simulink model "KheperaIV"  (R2020b)
settings: Solver=VariableStepAuto  StartTime=0.0  StopTime=10.0  RelTol=1e-3
undefined symbols (not defined in the file): I, kb, kt, L, La, m, N, r, Ra, Rr
settings Model: Creator=FranciscoJose  LastModifiedBy=FranciscoJose

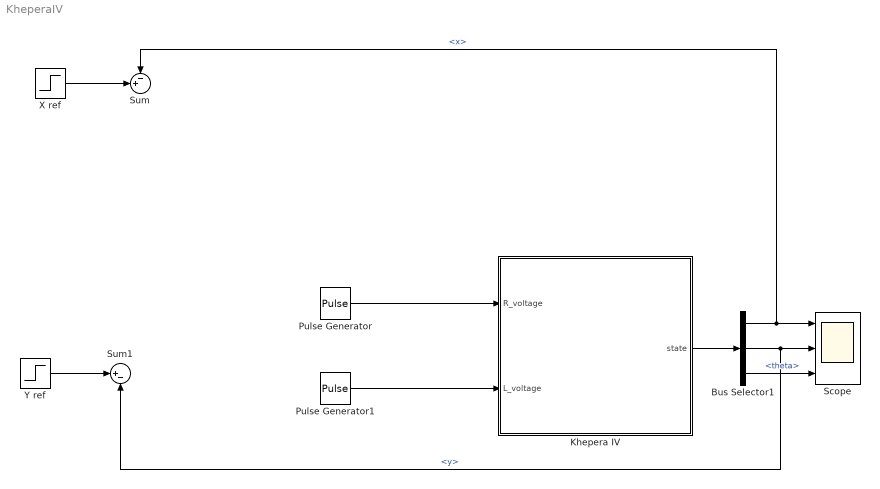
== system KheperaIV ==
  Bus Selector1 : BusSelector  OutputSignals=x,y,theta
  Khepera IV : Subsystem  mask{m=m, kb=kb, kt=kt, N=N, La=La, Ra=Ra, L=L, r=r, I=I, Rr=Rr}
      mask prompts: m "Mass [Kg]"; kb "Back-EMF constant [V/rad/s]"; kt "Torque constant [Nm/A]"; N "Gear ratio"; La "Rotor inductance [H]"; Ra "Terminal resistance [Ohm]"; L "Distance between wheels [m]"; r "Wheels radius [m]"; I "Moment inertia of robot [Kg m^2]"; Rr "Robot radius [m]"
      mask DialogControl DescTextVar Prompt: Khepera IV parameters
      mask Display: image('KheperaIV_icon.png')
  Pulse Generator : DiscretePulseGenerator  PulseType=Time based  Amplitude=6  Period=10  PulseWidth=10
  Pulse Generator1 : DiscretePulseGenerator  PulseType=Time based  Amplitude=-6  Period=10  PulseWidth=10
  Scope : Scope  NumInputPorts=3
  Sum : Sum  Inputs=-+|
  Sum1 : Sum  Inputs=|+-
  X ref : Step  SampleTime=0
  Y ref : Step  SampleTime=0
  wires:
  Khepera IV/1(state) -> Bus Selector1/1
  Bus Selector1/3 -> Scope/3  "<theta>"
  Bus Selector1/2 -> Scope/2, Sum1/2  "<y>"
  Bus Selector1/1 -> Sum/1, Scope/1  "<x>"
  Pulse Generator1/1 -> Khepera IV/2(L_voltage)
  Pulse Generator/1 -> Khepera IV/1(R_voltage)
  X ref/1 -> Sum/2
  Y ref/1 -> Sum1/1

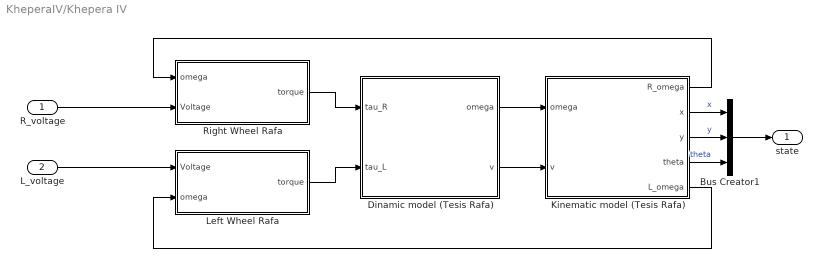
== system KheperaIV/Khepera IV ==
  R_voltage : Inport
  L_voltage : Inport  Port=2
  Bus Creator1 : BusCreator  Inputs=3
  Dinamic model (Tesis Rafa) : Subsystem
  Kinematic model (Tesis Rafa) : Subsystem
  Left Wheel Rafa : Subsystem
  Right Wheel Rafa : Subsystem
  state : Outport
  wires:
  L_voltage/1 -> Left Wheel Rafa/1(Voltage)
  R_voltage/1 -> Right Wheel Rafa/2(Voltage)
  Dinamic model (Tesis Rafa)/1(omega) -> Kinematic model (Tesis Rafa)/1(omega)
  Dinamic model (Tesis Rafa)/2(v) -> Kinematic model (Tesis Rafa)/2(v)
  Left Wheel Rafa/1(torque) -> Dinamic model (Tesis Rafa)/2(tau_L)
  Right Wheel Rafa/1(torque) -> Dinamic model (Tesis Rafa)/1(tau_R)
  Kinematic model (Tesis Rafa)/1(R_omega) -> Right Wheel Rafa/1(omega)
  Kinematic model (Tesis Rafa)/5(L_omega) -> Left Wheel Rafa/2(omega)
  Kinematic model (Tesis Rafa)/2(x) -> Bus Creator1/1  "x"
  Kinematic model (Tesis Rafa)/3(y) -> Bus Creator1/2  "y"
  Kinematic model (Tesis Rafa)/4(theta) -> Bus Creator1/3  "theta"
  Bus Creator1/1 -> state/1

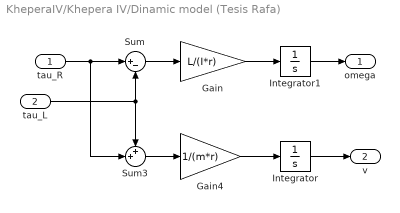
== system KheperaIV/Khepera IV/Dinamic model (Tesis Rafa) ==
  tau_R : Inport
  tau_L : Inport  Port=2
  Gain : Gain  Gain=L/(I*r)
  Gain4 : Gain  Gain=1/(m*r)
  Integrator : Integrator
  Integrator1 : Integrator
  Sum : Sum  Inputs=|+-
  Sum3 : Sum  Inputs=++|
  omega : Outport
  v : Outport  Port=2
  wires:
  Sum/1 -> Gain/1
  Integrator/1 -> v/1
  tau_R/1 -> Sum3/2, Sum/1
  Integrator1/1 -> omega/1
  Gain/1 -> Integrator1/1
  tau_L/1 -> Sum3/1, Sum/2
  Sum3/1 -> Gain4/1
  Gain4/1 -> Integrator/1

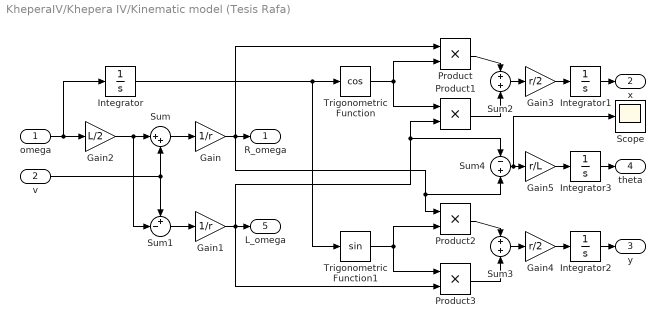
== system KheperaIV/Khepera IV/Kinematic model (Tesis Rafa) ==
  omega : Inport
  v : Inport  Port=2
  Gain : Gain  Gain=1/r
  Gain1 : Gain  Gain=1/r
  Gain2 : Gain  Gain=L/2
  Gain3 : Gain  Gain=r/2
  Gain4 : Gain  Gain=r/2
  Gain5 : Gain  Gain=r/L
  Integrator{,1..3} (4 alike) : Integrator
  Product{,1..3} (4 alike) : Product
  Scope : Scope
  Sum : Sum  Inputs=|++
  Sum1 : Sum  Inputs=+-|
  Sum2 : Sum
  Sum3 : Sum
  Sum4 : Sum  Inputs=-+
  Trigonometric Function : Trigonometry  Operator=cos
  Trigonometric Function1 : Trigonometry
  R_omega : Outport
  x : Outport  Port=2
  y : Outport  Port=3
  theta : Outport  Port=4
  L_omega : Outport  Port=5
  wires:
  Sum/1 -> Gain/1
  Gain2/1 -> Sum1/2, Sum/1
  v/1 -> Sum1/1, Sum/2
  Sum1/1 -> Gain1/1
  omega/1 -> Integrator/1, Gain2/1
  Gain3/1 -> Integrator1/1
  Integrator/1 -> Trigonometric Function1/1, Trigonometric Function/1
  Sum2/1 -> Gain3/1
  Product/1 -> Sum2/1
  Trigonometric Function/1 -> Product/2, Product1/1
  Product1/1 -> Sum2/2
  Gain/1 -> R_omega/1, Sum4/2, Product2/1, Product/1
  Trigonometric Function1/1 -> Product2/2, Product3/1
  Product3/1 -> Sum3/2
  Sum3/1 -> Gain4/1
  Gain1/1 -> L_omega/1, Product3/2, Sum4/1, Product1/2
  Product2/1 -> Sum3/1
  Integrator1/1 -> x/1
  Gain4/1 -> Integrator2/1
  Integrator2/1 -> y/1
  Integrator3/1 -> theta/1
  Gain5/1 -> Integrator3/1
  Sum4/1 -> Scope/1, Gain5/1

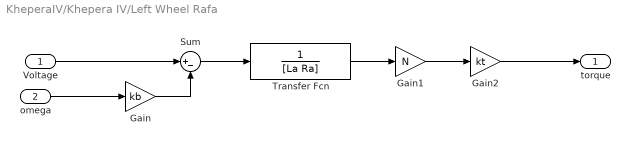
== system KheperaIV/Khepera IV/Left Wheel Rafa ==
  Voltage : Inport
  omega : Inport  Port=2
  Gain : Gain  Gain=kb
  Gain1 : Gain  Gain=N
  Gain2 : Gain  Gain=kt
  Sum : Sum  Inputs=|+-
  Transfer Fcn : TransferFcn  Denominator=[La Ra]
  torque : Outport
  wires:
  Transfer Fcn/1 -> Gain1/1
  Gain1/1 -> Gain2/1
  Gain/1 -> Sum/2
  Voltage/1 -> Sum/1
  Sum/1 -> Transfer Fcn/1
  Gain2/1 -> torque/1
  omega/1 -> Gain/1

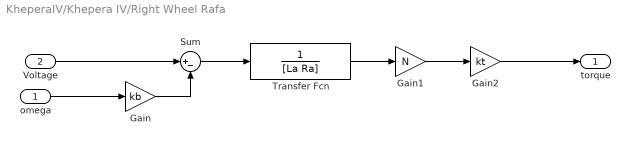
== system KheperaIV/Khepera IV/Right Wheel Rafa ==
  omega : Inport
  Voltage : Inport  Port=2
  Gain : Gain  Gain=kb
  Gain1 : Gain  Gain=N
  Gain2 : Gain  Gain=kt
  Sum : Sum  Inputs=|+-
  Transfer Fcn : TransferFcn  Denominator=[La Ra]
  torque : Outport
  wires:
  Transfer Fcn/1 -> Gain1/1
  Gain1/1 -> Gain2/1
  Gain/1 -> Sum/2
  Voltage/1 -> Sum/1
  Sum/1 -> Transfer Fcn/1
  Gain2/1 -> torque/1
  omega/1 -> Gain/1
